simulink model "mag_schwebe_fuzzy"  (Simulink 4.00)
settings: Solver=ode45  StartTime=0.0  StopTime=20.0  MaxStep=0.01  RelTol=1e-3
libraries: simulink3 x2, fuzblock x1
settings Model: LastModifiedBy=Brunner  MaxDataPoints=2000  BlockReductionOpt=off

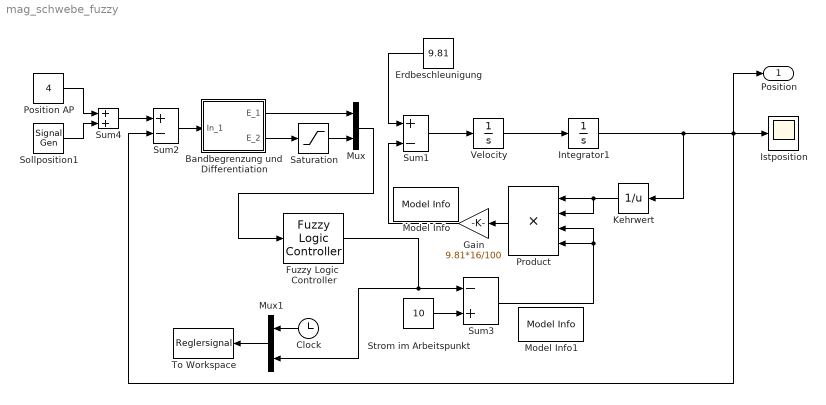
== system mag_schwebe_fuzzy ==
  Bandbegrenzung und Differentiation : Subsystem  mask(PID Controller){T0=0.1, T=0.01}
      mask prompts: T0 "Filter-Zeitkonstante"; T "Abtastintervall"
      mask help:
      | Enter expressions for proportional, integral, and derivative terms.
      | P+I/s+Ds
      settings: RTWFcnNameOpts=Auto  RTWFileNameOpts=Auto
      mask Help: This block implements a PID controller where parameters are entered for the Proportional, Integral and Derivative terms. Unmask this block to see how it works. The derivative term is implemented using a true derivative block.
      mask Display: disp('Digitalfilter')
  Clock : Clock
      settings: DisplayTime=off  Decimation=10
  Erdbeschleunigung : Constant  Orientation=left  Value=9.81
  Fuzzy Logic  Controller : fuzblock/Fuzzy Logic  Controller  fis='ball.fis'
  Gain : Gain  Orientation=left  Gain=9.81*16/100  Multiplication=Element-wise(K.*u)  SaturateOnIntegerOverflow=on
  Integrator1 : Integrator  ExternalReset=none  InitialConditionSource=internal  InitialCondition=4  LimitOutput=off  UpperSaturationLimit=inf  LowerSaturationLimit=-inf  ShowSaturationPort=off  ShowStatePort=off  AbsoluteTolerance=auto
  Istposition : Scope
      settings: TimeRange=20  YMin=3.93  YMax=4.08  SaveToWorkspace=off  SaveName=ScopeData  LimitDataPoints=on  MaxDataPoints=5000
  Kehrwert : Math  Orientation=left  Operator=reciprocal  OutputSignalType=auto
  Model Info : simulink3/Signals & Systems/Model Info  InitialBlockCM=none  BlockCM=none  Frame=off  DisplayStringWithTags=|  HorizontalTextAlignment=Center  LeftAlignmentValue=0.5  SourceBlockDiagram=mag_schwebe_fuzzy  TagMaxNumber=20
      | Magnet-
      | kraft (norm.)
  Model Info1 : simulink3/Signals & Systems/Model Info  InitialBlockCM=none  BlockCM=none  Frame=off  DisplayStringWithTags=geregelter Spulenstrom  HorizontalTextAlignment=Center  LeftAlignmentValue=0.5  SourceBlockDiagram=mag_schwebe_fuzzy  TagMaxNumber=20
  Mux : Mux  Inputs=2
  Mux1 : Mux  Orientation=left  Inputs=2
  Position AP : Constant  Value=4
  Product : Product  Orientation=left  Inputs=4  Multiplication=Element-wise(.*)  SaturateOnIntegerOverflow=on
  Saturation : Saturate  UpperLimit=0.5  LowerLimit=-0.5  LinearizeAsGain=on
  Sollposition1 : SignalGenerator  WaveForm=square  Amplitude=0.05  Frequency=0.1  Units=Hertz
  Strom im Arbeitspunkt : Constant  Value=10
  Sum1 : Sum  Inputs=+-  SaturateOnIntegerOverflow=on
  Sum2 : Sum  Inputs=+-  SaturateOnIntegerOverflow=on
  Sum3 : Sum  Inputs=-+  SaturateOnIntegerOverflow=on
  Sum4 : Sum  Inputs=++  SaturateOnIntegerOverflow=on
  To Workspace : ToWorkspace  VariableName=Reglersignal  SampleTime=-1  SaveFormat=Array
  Velocity : Integrator  ExternalReset=none  InitialConditionSource=internal  InitialCondition=0  LimitOutput=off  UpperSaturationLimit=inf  LowerSaturationLimit=-inf  ShowSaturationPort=off  ShowStatePort=off  AbsoluteTolerance=auto
  Position : Outport  Port=1
  wires:
  Gain/1 -> Sum1/2
  Sum1/1 -> Velocity/1
  Velocity/1 -> Integrator1/1
  Integrator1/1 -> Kehrwert/1, Istposition/1, Sum2/2, Position/1
  Product/1 -> Gain/1
  Kehrwert/1 -> Product/1, Product/2
  Position AP/1 -> Sum4/1
  Sollposition1/1 -> Sum4/2
  Erdbeschleunigung/1 -> Sum1/1
  Sum4/1 -> Sum2/1
  Sum2/1 -> Bandbegrenzung und Differentiation/1(In_1)
  Strom im Arbeitspunkt/1 -> Sum3/2
  Sum3/1 -> Product/3, Product/4
  Fuzzy Logic  Controller/1 -> Sum3/1, Mux1/2
  Mux1/1 -> To Workspace/1
  Clock/1 -> Mux1/1
  Bandbegrenzung und Differentiation/2(E_2) -> Saturation/1
  Bandbegrenzung und Differentiation/1(E_1) -> Mux/1
  Saturation/1 -> Mux/2
  Mux/1 -> Fuzzy Logic  Controller/1

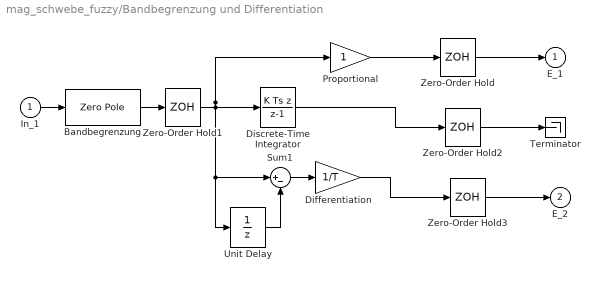
== system mag_schwebe_fuzzy/Bandbegrenzung und Differentiation ==
  In_1 : Inport  Port=1
  Bandbegrenzung : ZeroPole  Zeros=[]  Poles=[-1/T0]  Gain=[1/T0]  AbsoluteTolerance=auto
  Differentiation : Gain  Gain=1/T  Multiplication=Element-wise(K.*u)  SaturateOnIntegerOverflow=on
  Discrete-Time Integrator : DiscreteIntegrator  IntegratorMethod=BackwardEuler  ExternalReset=none  InitialConditionSource=internal  InitialCondition=0  LimitOutput=off  UpperSaturationLimit=inf  LowerSaturationLimit=-inf  ShowSaturationPort=off  ShowStatePort=off  SampleTime=T
  Proportional : Gain  Gain=1  Multiplication=Element-wise(K.*u)  SaturateOnIntegerOverflow=on
  Sum1 : Sum  Inputs=|+-  SaturateOnIntegerOverflow=on
  Terminator : Terminator
  Unit Delay : UnitDelay  X0=0  SampleTime=0.01
  Zero-Order Hold{,1..3} (4 alike) : ZeroOrderHold  SampleTime=T
  E_1 : Outport  Port=1  InitialOutput=0
  E_2 : Outport  Port=2  InitialOutput=0
  wires:
  In_1/1 -> Bandbegrenzung/1
  Bandbegrenzung/1 -> Zero-Order Hold1/1
  Zero-Order Hold/1 -> E_1/1
  Zero-Order Hold1/1 -> Discrete-Time Integrator/1, Proportional/1, Sum1/1, Unit Delay/1
  Sum1/1 -> Differentiation/1
  Unit Delay/1 -> Sum1/2
  Proportional/1 -> Zero-Order Hold/1
  Discrete-Time Integrator/1 -> Zero-Order Hold2/1
  Zero-Order Hold2/1 -> Terminator/1
  Zero-Order Hold3/1 -> E_2/1
  Differentiation/1 -> Zero-Order Hold3/1
